simulink model "CelulaFabricacionFlexible_Inicial"  (R2019b)
settings: Solver=VariableStepAuto  StartTime=0.0  StopTime=Inf  RelTol=1e-3
settings Model: EnablePacing=on  Creator=corsino  LastModifiedBy=Carlos

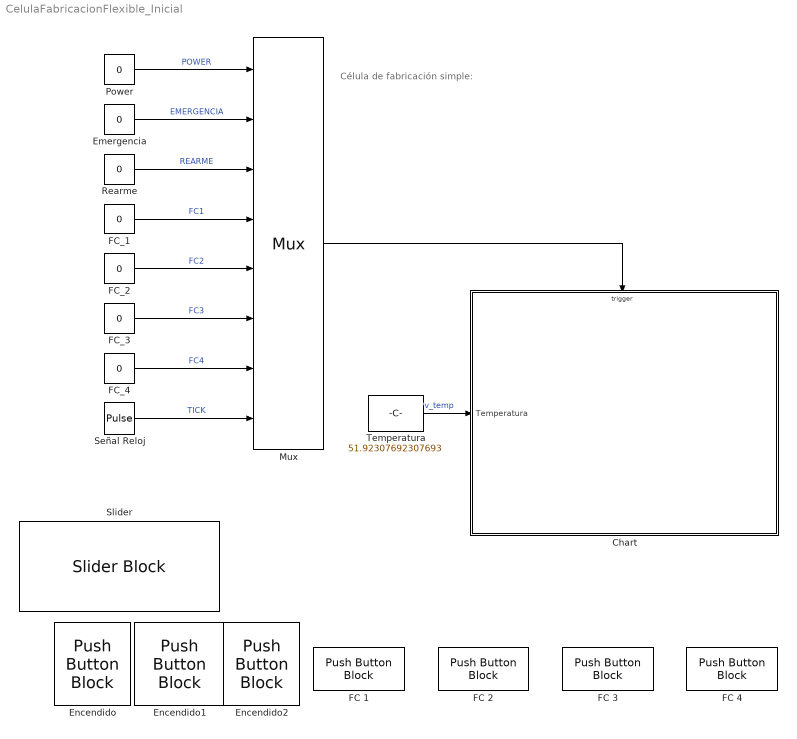
== system CelulaFabricacionFlexible_Inicial ==
  note: Célula de fabricación simple:
  Chart : Stateflow chart  BlockKeywords=__PRM__SERIALIZED__DATA__:Stateflow Chart,Stateflow Diagram  TreatAsAtomicUnit=on
  Emergencia : Constant  Value=0
  Encendido : PushButtonBlock  LabelPosition=Top  ButtonText=POWER
  Encendido1 : PushButtonBlock  LabelPosition=Top  ButtonText=EMERG.
  Encendido2 : PushButtonBlock  LabelPosition=Top  ButtonText=REARME
  FC 1 : PushButtonBlock  ButtonText=FC 1
  FC 2 : PushButtonBlock  ButtonText=FC 2
  FC 3 : PushButtonBlock  ButtonText=FC 3
  FC 4 : PushButtonBlock  ButtonText=FC 4
  FC_{1..4} (4 alike) : Constant  Value=0
  Mux : Mux  Inputs=8
      settings: DisplayOption=signals
  Power : Constant  Value=0
  Rearme : Constant  Value=0
  Señal Reloj : DiscretePulseGenerator  PulseType=Time based  Period=0.5  PulseWidth=50
  Slider : SliderBlock  ScaleMin=10  ScaleMax=60  TickInterval=5
  "Temperatura " : Constant  Value=51.92307692307693
  wires:
  FC_4/1 -> Mux/7  "FC4"
  FC_3/1 -> Mux/6  "FC3"
  FC_2/1 -> Mux/5  "FC2"
  FC_1/1 -> Mux/4  "FC1"
  Emergencia/1 -> Mux/2  "EMERGENCIA"
  Power/1 -> Mux/1  "POWER"
  Mux/1 -> Chart/Trigger
  "Temperatura "/1 -> Chart/1(Temperatura)  "v_temp"
  Señal Reloj/1 -> Mux/8  "TICK"
  Rearme/1 -> Mux/3  "REARME"

== stateflow chart CelulaFabricacionFlexible_Inicial/Chart ==
  settings: executeAtInitialization=1  initializeOutput=1
  state E_Encendido
    entry:
    Referencia = 35;
    TempHisteresis = 5;
    state E_Ciclo [parallel]
      settings: executionOrder=1
      state E_OP1
      state E_OP2
      state E_OP4
      state E_OP3
      (default) -> E_OP1
      E_OP1 -> E_OP2 : EV_FC1
      E_OP4 -> E_OP1 : EV_FC4
      E_OP2 -> E_OP3 : EV_FC2
      E_OP3 -> E_OP4 : EV_FC3
    state E_Ventilador [parallel]
      settings: executionOrder=2
      state E_Vent_off
      state E_Vent_on
      (default) -> E_Vent_off
      E_Vent_off -> E_Vent_on : EV_TICK[Temperatura>=(Referencia+TempHisteresis)]
      E_Vent_on -> E_Vent_off : EV_TICK[Temperatura<=(Referencia-TempHisteresis)]
  state E_Apagado
  state E_Error
  E_Apagado -> E_Encendido : EV_POWER
  E_Encendido -> E_Apagado [order 2] : EV_POWER
  E_Encendido -> E_Error [order 1] : EV_EMERGENCIA
  (default) -> E_Apagado
  E_Error -> E_Apagado : EV_REARME
  data: Temperatura input; Referencia local; TempHisteresis local
  events: EV_POWER input RISING_EDGE_EVENT; EV_EMERGENCIA input RISING_EDGE_EVENT; EV_REARME input RISING_EDGE_EVENT; EV_FC1 input RISING_EDGE_EVENT; EV_FC2 input RISING_EDGE_EVENT; EV_FC3 input RISING_EDGE_EVENT; EV_FC4 input RISING_EDGE_EVENT; EV_TICK input RISING_EDGE_EVENT
